simulink model "FINAL_MLC_IPC"  (Simulink 9.2)
settings: Solver=ode4  StartTime=0.0  StopTime=Parameter.Time.TMax  FixedStep=Parameter.Time.dt  RelTol=1e-3  EnableMultiTasking=on
undefined symbols (not defined in the file or in its folder): OutList, Parameter, strmatch, x2_t0
libraries: simulink x13
(part 2 of 2)

== matlab function MLC_IPC/pitch_ctrl_1/integral_signal ==
  data: u input double; y output double
function y = fcn(u)
y = cos((((cos(((my_div((-6.021),(-4.139))) + ((-8.9) + (-2.656)))) * sin((my_log((-5.506)) + (9.254 - (-5.814))))) - (cos((cos(5.765) - (my_div(4.159,0.4555)))) + my_log(((my_div(u(2),u(26))) + cos((-7.49)))))) - sin((cos(my_log((6.198 + u(7)))) * cos(((u(46) + 2.414) - (my_div(6.975,5.819))))))));

== matlab function MLC_IPC/pitch_ctrl_2/direct_signal ==
  data: u input double; y output double
function y = fcn(u)
y = cos((((cos(((my_div((-6.021),(-4.139))) + ((-8.9) + (-2.656)))) * sin((my_log((-5.506)) + (9.254 - (-5.814))))) - (cos((cos(5.765) - (my_div(4.159,0.4555)))) + my_log(((my_div(u(2),u(26))) + cos((-7.49)))))) - sin((cos(my_log((6.198 + u(7)))) * cos(((u(46) + 2.414) - (my_div(6.975,5.819))))))));

== matlab function MLC_IPC/pitch_ctrl_2/integral_signal ==
  data: u input double; y output double
function y = fcn(u)
y = cos(((((my_div(((u(9) + 6.486) * sin((-0.8411))),my_log(cos(u(9))))) + (sin(my_log((-6.301))) - ((u(26) + u(47)) - sin((-4.179))))) * (my_div(((sin((-6.813)) * my_log((-2.407))) + (cos(4.909) + sin(6.878))),cos((((-3.952) - u(34)) - (u(5) - u(47))))))) + my_log(((cos(sin(u(9))) - my_log((u(10) + u(3)))) * (sin(((-0.07202) + 9.768)) * (my_div((u(34) + (-6.601)),(u(74) - u(7)))))))));

== matlab function MLC_IPC/pitch_ctrl_3/direct_signal ==
  data: u input double; y output double
function y = fcn(u)
y = my_log(cos(my_log(my_log(cos(my_log(my_log((-5.282))))))));

== matlab function MLC_IPC/pitch_ctrl_3/integral_signal ==
  data: u input double; y output double
function y = fcn(u)
y = sin(((((my_div(sin(sin((-1.594))),((u(91) - 7.727) * (4.836 + u(10))))) + my_log(cos((my_div((-4.663),(-9.273)))))) - sin((my_div((sin((-3.975)) - sin((-5.546))),sin((5.15 - (-5.354))))))) * ((my_div((cos((u(34) - 2.57)) - (cos(u(2)) + (u(91) * 6.704))),(((my_div(u(9),u(34))) + (5.097 - u(25))) + cos((my_div(u(9),(-9.534))))))) + (my_div(((((-9.381) - u(24)) + (u(3) - (-9.479))) * ((u(3) - (-6.724)) + (3.95 * (-5.042)))),sin(((1.209 * 2.107) * sin(5.893))))))));
